simulink model "Check_my_EoM_for_Mac"  (R2020b)
settings: Solver=FixedStepAuto  StartTime=0.0  StopTime=95  FixedStep=CNT_StepSize  RelTol=1e-3
undefined symbols (not defined in the file or in its folder): CNT_StepSize
libraries: simulink x3
settings Model: Creator=NicolasS  LastModifiedBy=leifr

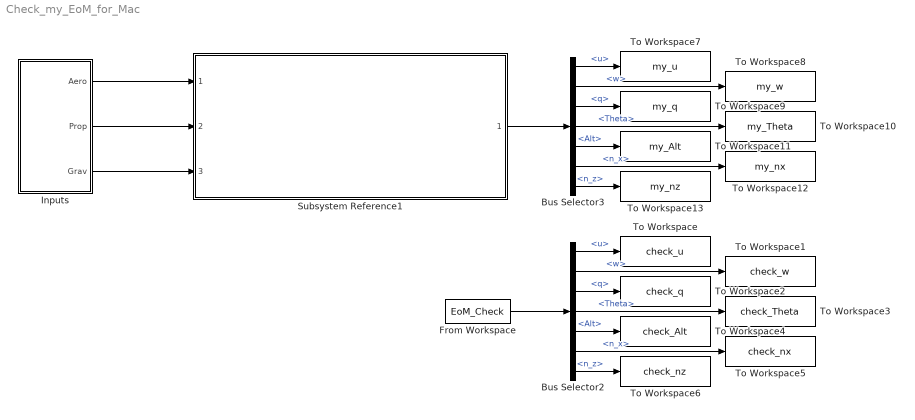
== system Check_my_EoM_for_Mac ==
  Bus Selector2 : BusSelector  OutputSignals=vv_f.u,vv_f.w,q,Theta,Alt,nn_f.n_x,nn_f.n_z
  Bus Selector3 : BusSelector  OutputSignals=vv_f.u,vv_f.w,q,Theta,Alt,nn_f.n_x,nn_f.n_z
  From Workspace : FromWorkspace  VariableName=EoM_Check  OutDataTypeStr=Bus: EoM  SampleTime=CNT_StepSize
  Inputs : Subsystem
  Subsystem Reference1 : Subsystem  ReferencedSubsystem=Equations_of_Motion
  To Workspace : ToWorkspace  VariableName=check_u  SaveFormat=Timeseries  SampleTime=-1
  To Workspace1 : ToWorkspace  VariableName=check_w  SaveFormat=Timeseries  SampleTime=-1
  To Workspace10 : ToWorkspace  VariableName=my_Theta  SaveFormat=Timeseries  SampleTime=-1
  To Workspace11 : ToWorkspace  VariableName=my_Alt  SaveFormat=Timeseries  SampleTime=-1
  To Workspace12 : ToWorkspace  VariableName=my_nx  SaveFormat=Timeseries  SampleTime=-1
  To Workspace13 : ToWorkspace  VariableName=my_nz  SaveFormat=Timeseries  SampleTime=-1
  To Workspace2 : ToWorkspace  VariableName=check_q  SaveFormat=Timeseries  SampleTime=-1
  To Workspace3 : ToWorkspace  VariableName=check_Theta  SaveFormat=Timeseries  SampleTime=-1
  To Workspace4 : ToWorkspace  VariableName=check_Alt  SaveFormat=Timeseries  SampleTime=-1
  To Workspace5 : ToWorkspace  VariableName=check_nx  SaveFormat=Timeseries  SampleTime=-1
  To Workspace6 : ToWorkspace  VariableName=check_nz  SaveFormat=Timeseries  SampleTime=-1
  To Workspace7 : ToWorkspace  VariableName=my_u  SaveFormat=Timeseries  SampleTime=-1
  To Workspace8 : ToWorkspace  VariableName=my_w  SaveFormat=Timeseries  SampleTime=-1
  To Workspace9 : ToWorkspace  VariableName=my_q  SaveFormat=Timeseries  SampleTime=-1
  wires:
  Bus Selector2/4 -> To Workspace3/1  "<Theta>"
  Bus Selector2/3 -> To Workspace2/1  "<q>"
  Bus Selector2/7 -> To Workspace6/1  "<n_z>"
  Bus Selector2/1 -> To Workspace/1  "<u>"
  Bus Selector2/2 -> To Workspace1/1  "<w>"
  Bus Selector2/6 -> To Workspace5/1  "<n_x>"
  Bus Selector2/5 -> To Workspace4/1  "<Alt>"
  Bus Selector3/5 -> To Workspace11/1  "<Alt>"
  Bus Selector3/6 -> To Workspace12/1  "<n_x>"
  Bus Selector3/2 -> To Workspace8/1  "<w>"
  Bus Selector3/1 -> To Workspace7/1  "<u>"
  Bus Selector3/7 -> To Workspace13/1  "<n_z>"
  Bus Selector3/3 -> To Workspace9/1  "<q>"
  Bus Selector3/4 -> To Workspace10/1  "<Theta>"
  Subsystem Reference1/1 -> Bus Selector3/1
  Inputs/1(Aero) -> Subsystem Reference1/1
  Inputs/2(Prop) -> Subsystem Reference1/2
  Inputs/3(Grav) -> Subsystem Reference1/3
  From Workspace/1 -> Bus Selector2/1

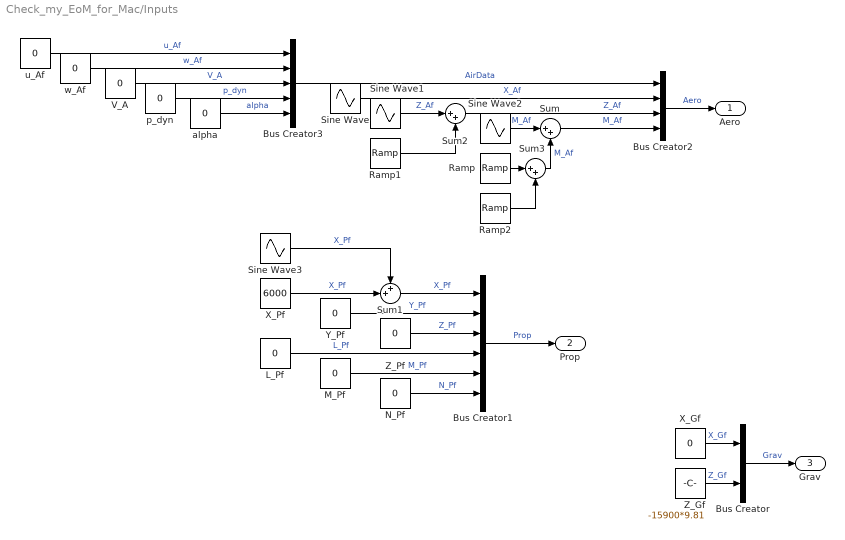
== system Check_my_EoM_for_Mac/Inputs ==
  Bus Creator : BusCreator  Inputs=2  OutDataTypeStr=Bus: Grav
  Bus Creator1 : BusCreator  Inputs=6  OutDataTypeStr=Bus: Prop
  Bus Creator2 : BusCreator  Inputs=4  OutDataTypeStr=Bus: Aero
  Bus Creator3 : BusCreator  Inputs=5  OutDataTypeStr=Bus: AirData
  L_Pf : Constant  Value=0  SampleTime=-1
  M_Pf : Constant  Value=0  SampleTime=-1
  N_Pf : Constant  Value=0  SampleTime=-1
  Ramp : simulink/Sources/Ramp  slope=-0.5  start=0  InitialOutput=0
  Ramp1 : simulink/Sources/Ramp  slope=75  start=75  InitialOutput=0
  Ramp2 : simulink/Sources/Ramp  slope=4  start=50  InitialOutput=0
  Sine Wave : Sin  Amplitude=500  Bias=-6000  Frequency=0.25  Phase=45  SampleTime=CNT_StepSize
  Sine Wave1 : Sin  Amplitude=500  Bias=155979  Frequency=0.4  SampleTime=CNT_StepSize
  Sine Wave2 : Sin  Amplitude=400  Frequency=0.7  Phase=-30  SampleTime=CNT_StepSize
  Sine Wave3 : Sin  Amplitude=1000  Frequency=0.2  Phase=75  SampleTime=CNT_StepSize
  Sum : Sum  Inputs=|++
  Sum1 : Sum  Inputs=++|
  Sum2 : Sum  Inputs=|++
  Sum3 : Sum  Inputs=|++
  V_A : Constant  Value=0  SampleTime=-1
  X_Gf : Constant  Value=0  SampleTime=-1
  X_Pf : Constant  Value=6000  SampleTime=-1
  Y_Pf : Constant  Value=0  SampleTime=-1
  Z_Gf : Constant  Value=-15900*9.81  SampleTime=-1
  Z_Pf : Constant  Value=0  SampleTime=-1
  alpha : Constant  Value=0  SampleTime=-1
  p_dyn : Constant  Value=0  SampleTime=-1
  u_Af : Constant  Value=0  SampleTime=-1
  w_Af : Constant  Value=0  SampleTime=-1
  Aero : Outport  OutDataTypeStr=Bus: Aero
  Prop : Outport  Port=2  OutDataTypeStr=Bus: Prop
  Grav : Outport  Port=3  OutDataTypeStr=Bus: Grav  SampleTime=[0.001,0]
  wires:
  Bus Creator2/1 -> Aero/1  "Aero"
  Z_Gf/1 -> Bus Creator/2  "Z_Gf"
  u_Af/1 -> Bus Creator3/1  "u_Af"
  Ramp2/1 -> Sum3/2
  Sum1/1 -> Bus Creator1/1  "X_Pf"
  Bus Creator/1 -> Grav/1  "Grav"
  M_Pf/1 -> Bus Creator1/5  "M_Pf"
  N_Pf/1 -> Bus Creator1/6  "N_Pf"
  alpha/1 -> Bus Creator3/5  "alpha"
  Sine Wave1/1 -> Sum2/1  "Z_Af"
  Sum2/1 -> Bus Creator2/3  "Z_Af"
  L_Pf/1 -> Bus Creator1/4  "L_Pf"
  w_Af/1 -> Bus Creator3/2  "w_Af"
  Z_Pf/1 -> Bus Creator1/3  "Z_Pf"
  Bus Creator1/1 -> Prop/1  "Prop"
  p_dyn/1 -> Bus Creator3/4  "p_dyn"
  X_Gf/1 -> Bus Creator/1  "X_Gf"
  X_Pf/1 -> Sum1/2  "X_Pf"
  Ramp1/1 -> Sum2/2
  Y_Pf/1 -> Bus Creator1/2  "Y_Pf"
  V_A/1 -> Bus Creator3/3  "V_A"
  Ramp/1 -> Sum3/1
  Sum/1 -> Bus Creator2/4  "M_Af"
  Bus Creator3/1 -> Bus Creator2/1  "AirData"
  Sine Wave3/1 -> Sum1/1  "X_Pf"
  Sum3/1 -> Sum/2  "M_Af"
  Sine Wave2/1 -> Sum/1  "M_Af"
  Sine Wave/1 -> Bus Creator2/2  "X_Af"
